simulink model "uwb_4_delay_mult_test"  (R2025a)
settings: Solver=VariableStepAuto  StartTime=0.0  StopTime=1e-7  RelTol=1e-3
libraries: dspfdesign x1, dspstat3 x1, commdigbbndpm3 x1, simulink x1
settings Model: Creator=IWMAI  LastModifiedBy=IWMAI

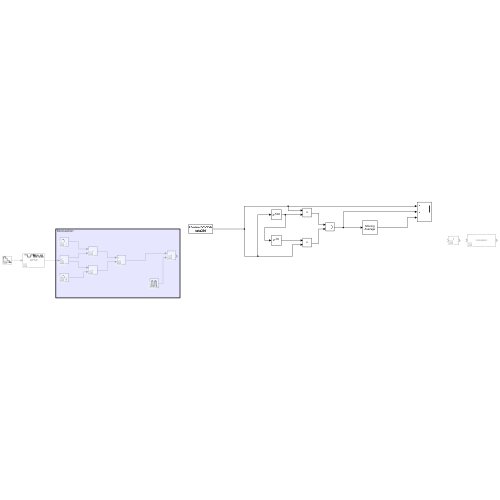
[thumbnail: Simulink's stored preview of the top-level diagram]
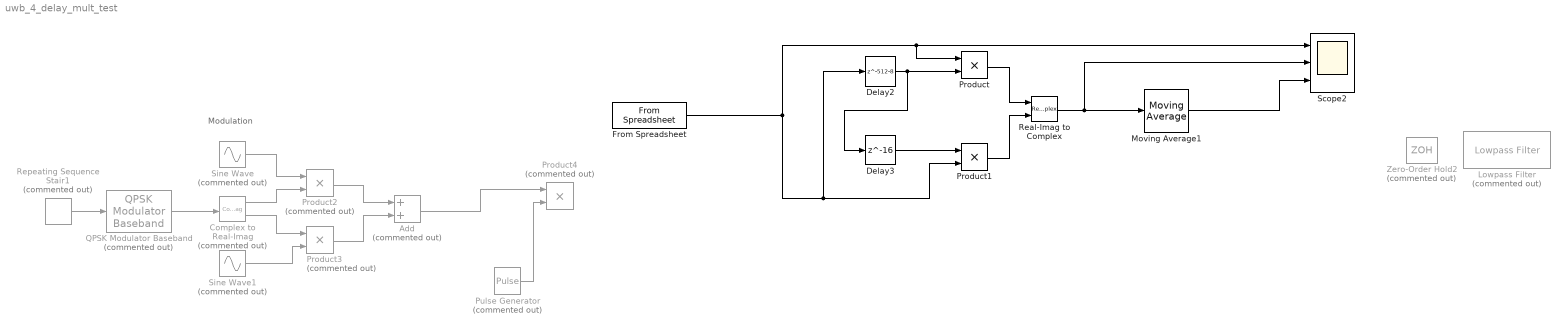
== system uwb_4_delay_mult_test ==
  note: Modulation
  Add : Sum  Commented=on
  Complex to Real-Imag : ComplexToRealImag  Commented=on
  Delay2 : Delay  DelayLength=512-8
  Delay3 : Delay  DelayLength=16
  From Spreadsheet : FromSpreadsheet  FileName=C:\Users\IWMAI\University of Toronto\Yu Huang - Summer-2025-sharted\Yongkang\v3_250617\csv\data256.csv  SheetName=data256  SampleTime=1/256e9
  Lowpass Filter : dspfdesign/Lowpass Filter  Commented=on  FilterType=FIR  DesignForMinimumOrder=on  FilterOrder=50  PassbandFrequency=1/128  StopbandFrequency=1/64  PassbandRipple=0.1  StopbandAttenuation=80  SampleRateMode=Use normalized frequency (0 to 1)  SampleRate=44100  SimulateUsing=Interpreted execution  roundingMode=Floor  coeffsDataTypeStr=fixdt(1,16)
  Moving Average1 : dspstat3/Moving Average  Method=Sliding window  ForgettingFactorPort=off  SpecifyWindowLength=on  WindowLength=256  OverlapLength=255  AllowArbitraryInputLength=off  ForgettingFactor=0.9  SimulateUsing=Interpreted execution
  Product : Product
  Product1 : Product
  Product2 : Product  Commented=on
  Product3 : Product  Commented=on
  Product4 : Product  Commented=on
  Pulse Generator : DiscretePulseGenerator  Commented=on  PulseType=Time based  Period=1/500e6  PulseWidth=37.5  PhaseDelay=1/256e9  SampleTime=0.000001
  QPSK Modulator Baseband : commdigbbndpm3/QPSK Modulator Baseband  Commented=on  InType=Integer  Enc=Binary  Ph=pi/4  outDtype=double  outWordLen=16  outUDDataType=sfix(16)  outFracLenMode=Best precision  outFracLen=15  outDataTypeStr=double  outLastDataTypeStr=double
      settings: LibrarySourceBlock=|
      | commhdldigbbndpm/QPSK
      | Modulator
      | Baseband
  Real-Imag to Complex : RealImagToComplex
  Repeating Sequence Stair1 : simulink/Sources/Repeating Sequence Stair  Commented=on  OutValues=[3 3 2 2 1 1 0 0].'  tsamp=1/500e6  OutMin=[]  OutMax=[]  OutDataTypeStr=double  OutputDataTypeScalingMode=double  OutDataType=fixdt(0,8)  ConRadixGroup=Best Precision: Vector-wise  OutScaling=2^-12
  Scope2 : Scope  NumInputPorts=3
      settings: ActiveDisplayYMinimum=-0.17970731877378929  ActiveDisplayYMaximum=0.16923044358029937  DataLoggingVariableName=ScopeData2
  Sine Wave : Sin  Commented=on  Frequency=2*pi*4e9  Phase=pi/2  SampleTime=1/256e9
  Sine Wave1 : Sin  Commented=on  Frequency=2*pi*4e9  SampleTime=1/256e9
  Zero-Order Hold2 : ZeroOrderHold  Commented=on  SampleTime=-1
  wires:
  Delay2/1 -> Delay3/1, Product/2
  Delay3/1 -> Product1/1
  Product/1 -> Real-Imag to Complex/1
  Product1/1 -> Real-Imag to Complex/2
  Real-Imag to Complex/1 -> Moving Average1/1, Scope2/2
  Moving Average1/1 -> Scope2/3
  Pulse Generator/1 -> Product4/2
  Complex to Real-Imag/2 -> Product3/1
  Product3/1 -> Add/2
  Sine Wave1/1 -> Product3/2
  Add/1 -> Product4/1
  Complex to Real-Imag/1 -> Product2/2
  Product2/1 -> Add/1
  Sine Wave/1 -> Product2/1
  Repeating Sequence Stair1/1 -> QPSK Modulator Baseband/1
  From Spreadsheet/1 -> Delay2/1, Product1/2, Product/1, Scope2/1
  QPSK Modulator Baseband/1 -> Complex to Real-Imag/1
